simulink model "Aufgabe_4_3_1_Einfache_systeme"  (R2024a)
settings: Solver=ode3  StartTime=0.0  StopTime=10.0  RelTol=1e-3
settings Model: Creator=ASUS  LastModifiedBy=ASUS

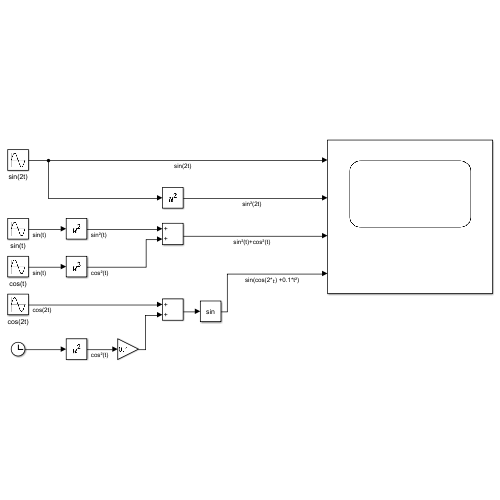
[thumbnail: Simulink's stored preview of the top-level diagram]
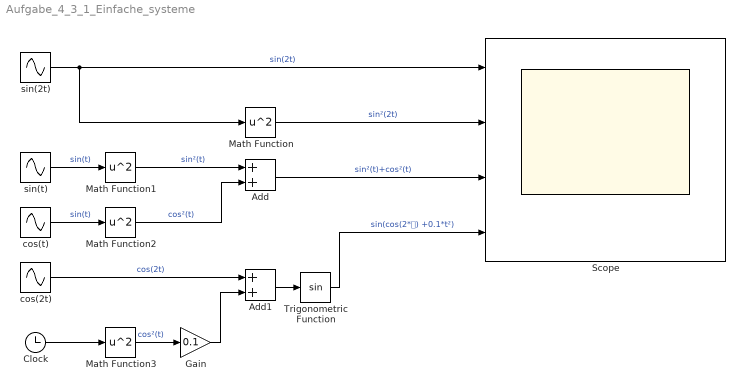
== system Aufgabe_4_3_1_Einfache_systeme ==
  Add : Sum
  Add1 : Sum
  Clock : Clock
  Gain : Gain  Gain=0.1
  Math Function{,1..3} (4 alike) : Math  Operator=square
  Scope : Scope  NumInputPorts=4
  Trigonometric Function : Trigonometry
  cos(2t) : Sin  Frequency=2  Phase=pi/2  SampleTime=0
  cos(t) : Sin  Phase=pi/2  SampleTime=0
  sin(2t) : Sin  Frequency=2  SampleTime=0
  sin(t) : Sin  SampleTime=0
  wires:
  sin(2t)/1 -> Math Function/1, Scope/1  "sin(2t)"
  Math Function/1 -> Scope/2  "sin²(2t)"
  sin(t)/1 -> Math Function1/1  "sin(t)"
  cos(t)/1 -> Math Function2/1  "sin(t)"
  Math Function1/1 -> Add/1  "sin²(t)"
  Math Function2/1 -> Add/2  "cos²(t)"
  Add/1 -> Scope/3  "sin²(t)+cos²(t)"
  Clock/1 -> Math Function3/1
  Math Function3/1 -> Gain/1  "cos²(t)"
  cos(2t)/1 -> Add1/1  "cos(2t)"
  Gain/1 -> Add1/2
  Add1/1 -> Trigonometric Function/1
  Trigonometric Function/1 -> Scope/4  "sin(cos(2*𝑡) +0.1*t²)"
